simulink model "RM3_Hydraulic_PTO"  (R2019b)
settings: Solver=ode14x  StartTime=0  StopTime=100  FixedStep=0.0025  MaxStep=0.0025  RelTol=1e-3  EnableMultiTasking=on
undefined symbols (not defined in the file or in its folder): body, DiscIntNeverNeededParam, pto
libraries: fl_lib x208, sh_lib x67, nesl_utility x67, WECSim_Lib x5
(part 1 of 5)
settings Model: Creator=mlawson  LastModifiedBy=remil
settings SolverCC: ZeroCrossControl=DisableAll  AlgebraicLoopSolver=LineSearch  AutoInsertRateTranBlk=on
settings DataIOCC: SaveFormat=Array  SaveOutput=off  SaveTime=off  ReturnWorkspaceOutputs=off
settings OptimizationCC: LifeSpan=inf  SimCompilerOptimization=on
settings DebuggingCC: UnderspecifiedInitializationDetection=Classic  MergeDetectMultiDrivingBlocksExec=none  SolverPrmCheckMsg=warning  AllowSymbolicDim=off  StateNameClashWarn=warning  SFUnexpectedBacktrackingDiag=warning  SFNoUnconditionalDefaultTransitionDiag=warning  ArithmeticOperatorsInVariantConditions=warning
settings HardwareCC: ProdBitPerPointer=32  ProdBitPerSizeT=32  ProdBitPerPtrDiffT=32  ProdLargestAtomicFloat=None  ProdIntDivRoundTo=Undefined  ProdEndianess=Unspecified  ProdWordSize=32  ProdHWDeviceType=32-bit Generic
settings ModelReferenceCC: PropagateSignalLabelsOutOfModel=off
settings SFSimCC: SimUseLocalCustomCode=off  CustomCodeUndefinedFunction=UseInterfaceOnly
settings RTWCC: RTWUseLocalCustomCode=off
settings CodeAppCC: StateflowObjectComments=on
settings GRTTargetCC: TargetLangStandard=C89/C90 (ANSI)  GeneratePreprocessorConditionals=Disable all
settings ConfigComp: CovMetricSettings=dw  CovHtmlReporting=on  CovSaveCumulativeToWorkspaceVar=on  CovSaveSingleToWorkspaceVar=on  CovExternalEMLEnable=off  CovSFcnEnable=off
settings SimscapeCC: SimscapeNormalizeSystem=off  SimscapeLogType=all  SimscapeLogSimulationStatistics=on  SimscapeLogOpenViewer=on
settings SimMechanicsCC: VisDuringSimulation=on
settings ExplorerConfigSet: SimMechanicsOpenEditorOnUpdate=off

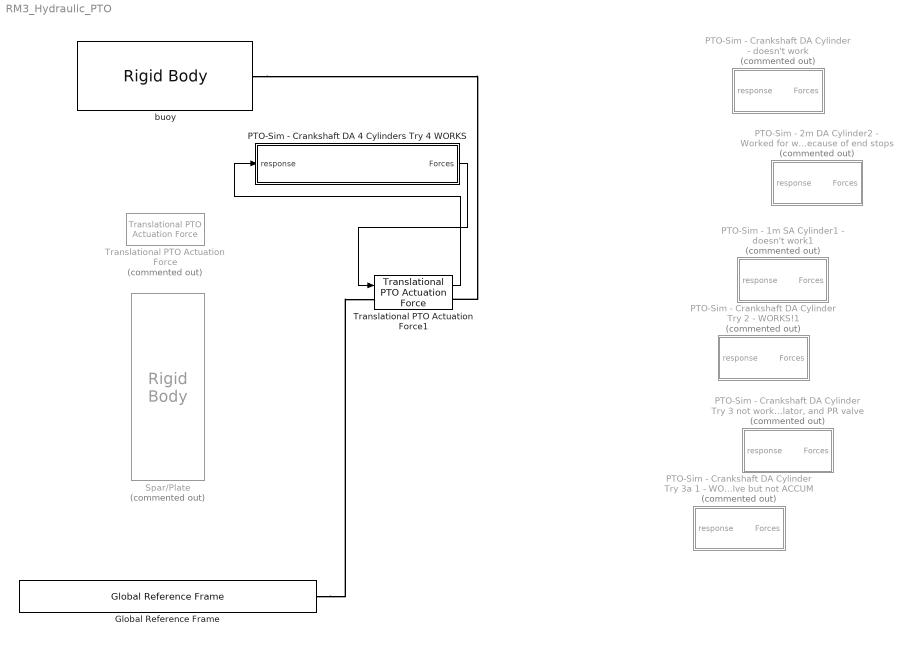
== system RM3_Hydraulic_PTO ==
  Global Reference Frame : WECSim_Lib/Frames/Global Reference Frame  waves=waves  simu=simu
      settings: SourceProductName=WEC-Sim
  PTO-Sim - 1m SA Cylinder1 - doesn't work1 : Subsystem  Commented=on
  "PTO-Sim - 2m DA Cylinder2 - Worked for waves up to 2m then forces go to infinity because of end stops   " : Subsystem  Commented=on
  "PTO-Sim - Crankshaft DA 4 Cylinders Try 4 WORKS " : Subsystem
  PTO-Sim - Crankshaft DA Cylinder - doesn't work : Subsystem  Commented=on
  PTO-Sim - Crankshaft DA Cylinder Try 2 - WORKS!1 : Subsystem  Commented=on
  "PTO-Sim - Crankshaft DA Cylinder Try 3 not working1 - added in correct PTO Force calculation, accumulator, and PR valve" : Subsystem  Commented=on
  PTO-Sim - Crankshaft DA Cylinder Try 3a 1 - WORKS - with PR valve but not ACCUM : Subsystem  Commented=on
  Spar/Plate : WECSim_Lib/Body Elements/Rigid Body  Commented=on  body=body(2)
      settings: AttributesFormatString=%<body>  SourceProductName=WEC-Sim
  Translational PTO Actuation Force : WECSim_Lib/PTOs/Translational PTO Actuation Force  Commented=on  pto=pto(1)
      settings: AttributesFormatString=%<pto>  SourceProductName=WEC-Sim
  Translational PTO Actuation Force1 : WECSim_Lib/PTOs/Translational PTO Actuation Force  pto=pto(1)
      settings: AttributesFormatString=%<pto>  SourceProductName=WEC-Sim
  buoy : WECSim_Lib/Body Elements/Rigid Body  body=body(1)
      settings: AttributesFormatString=%<body>  SourceProductName=WEC-Sim
  wires:
  "PTO-Sim - Crankshaft DA 4 Cylinders Try 4 WORKS "/1(Forces) -> Translational PTO Actuation Force1/1
  Translational PTO Actuation Force1/1 -> "PTO-Sim - Crankshaft DA 4 Cylinders Try 4 WORKS "/1(response)
  connections:
  buoy/RConn1 -- Translational PTO Actuation Force1/RConn1
  Global Reference Frame/RConn1 -- Translational PTO Actuation Force1/LConn1

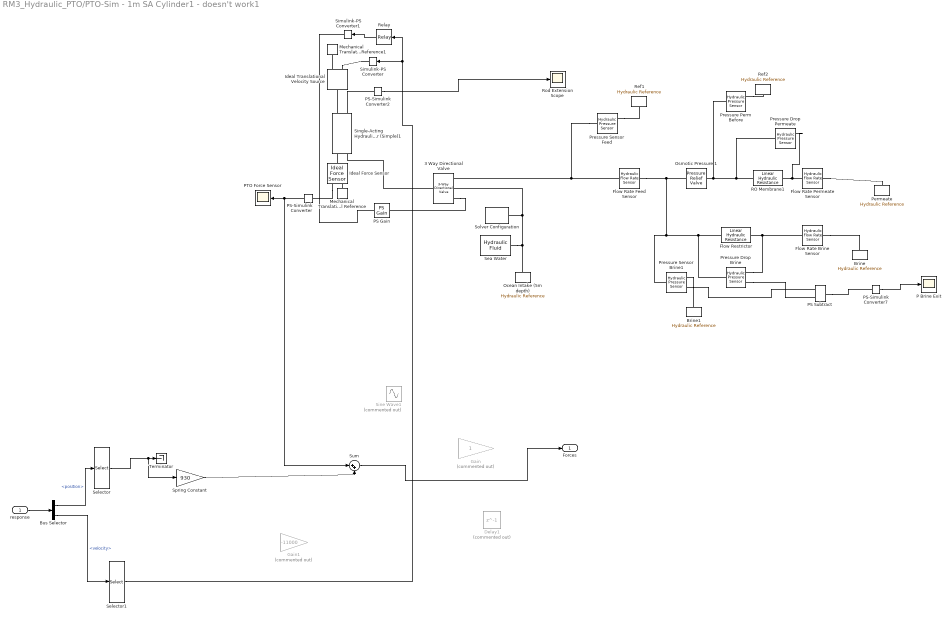
== system RM3_Hydraulic_PTO/PTO-Sim - 1m SA Cylinder1 - doesn't work1 ==
  response : Inport
  " Flow Rate Feed Sensor" : fl_lib/Hydraulic/Hydraulic Sensors/Hydraulic Flow Rate Sensor
      settings: SourceProductName=Simscape
  3 Way Directional Valve : sh_lib/Valves/Directional Valves/3-Way Directional Valve  area_spec=sh.valves.directional_valves.enum.area_spec.identical  x_0_P=0 m  x_0_T=0 m  mdl_type_identical=sh.valves.directional_valves.enum.mdl_type.linear  mdl_type_different=sh.valves.directional_valves.enum.mdl_type.linear  opening_max=0.75 in  area_max=pi*(0.75/2)^2 in^2  opening_max_P_A=0.005 m  area_max_P_A=0.5e-4 m^2  opening_max_A_T=0.005 m  area_max_A_T=0.5e-4 m^2  opening_area_tab=[-.002, 0, .002, .005, .015] m  area_tab=[1e-09, 2.0352e-07, 4.0736e-05, .00011438, .00034356] m^2  opening_flow_rate_tab=[-.002, 0, .002, .005, .015] m  pressure_tab=[-10000000, -5000000, -2000000, 2000000, 5000000, 10000000] Pa  flow_rate_tab=[-1e-07, -7.0711e-08, -4.4721e-08, 4.4721e-08, 7.0711e-08, 1e-07; -2.0352e-05, -1.4391e-05, -9.1017e-06, 9.1017e-06, 1.4391e-05, 2.0352e-05; -.0040736, -.0028805, -.0018218, .0018218, .0028805, .0040736; -.011438, -.0080879, -.0051152, .0051152, .0080879, .011438; -.034356, -.024293, -.015364, .015364, .024293, .034356] m^3/s  opening_area_tab_P_A=[-.002, 0, .002, .005, .015] m  area_tab_P_A=[1e-09, 2.0352e-07, 4.0736e-05, .00011438, .00034356] m^2  opening_flow_rate_tab_P_A=[-.002, 0, .002, .005, .015] m  pressure_tab_P_A=[-10000000, -5000000, -2000000, 2000000, 5000000, 10000000] Pa  flow_rate_tab_P_A=[-1e-07, -7.0711e-08, -4.4721e-08, 4.4721e-08, 7.0711e-08, 1e-07; -2.0352e-05, -1.4391e-05, -9.1017e-06, 9.1017e-06, 1.4391e-05, 2.0352e-05; -.0040736, -.0028805, -.0018218, .0018218, .0028805, .0040736; -.011438, -.0080879, -.0051152, .0051152, .0080879, .011438; -.034356, -.024293, -.015364, .015364, .024293, .034356] m^3/s  opening_area_tab_A_T=[-.002, 0, .002, .005, .015] m  area_tab_A_T=[1e-09, 2.0352e-07, 4.0736e-05, .00011438, .00034356] m^2  opening_flow_rate_tab_A_T=[-.002, 0, .002, .005, .015] m  pressure_tab_A_T=[-10000000, -5000000, -2000000, 2000000, 5000000, 10000000] Pa  flow_rate_tab_A_T=[-1e-07, -7.0711e-08, -4.4721e-08, 4.4721e-08, 7.0711e-08, 1e-07; -2.0352e-05, -1.4391e-05, -9.1017e-06, 9.1017e-06, 1.4391e-05, 2.0352e-05; -.0040736, -.0028805, -.0018218, .0018218, .0028805, .0040736; -.011438, -.0080879, -.0051152, .0051152, .0080879, .011438; -.034356, -.024293, -.015364, .015364, .024293, .034356] m^3/s  interp_method_identical=sh.valves.directional_valves.enum.interp_method.linear  interp_method_different=sh.valves.directional_valves.enum.interp_method.linear  extrap_method_identical=sh.valves.directional_valves.enum.extrap_method.linear  extrap_method_different=sh.valves.directional_valves.enum.extrap_method.linear  A_leak=1e-12 m^2  C_d=0.7  lam_spec=sh.valves.directional_valves.enum.lam_spec.pressure_ratio  B_lam=0.999  Re_cr=12
      settings: SourceProductName=Simscape Fluids  SourceProductBaseCode=SH  InternalSimscapePortConfiguration="{\"Bottom\":[],\"Left\":[{\"id\":\"A\",\"label\":\"A\",\"type\":\"foundation.hydraulic.hydraulic\"}],\"Right\":[{\"id\":\"S\",\"label\":\"S\",\"type\":\"input\"},{\"id\":\"P\",\"label\":\"P\",\"type\":\"foundation.hydraulic.hydraulic\"},{\"id\":\"T\",\"label\":\"T\",\"type\":\"foundation.hydraulic.hydraulic\"}],\"Top\":[]}"
  Brine : fl_lib/Hydraulic/Hydraulic Elements/Hydraulic Reference
      settings: SourceProductName=Simscape
  Brine1 : fl_lib/Hydraulic/Hydraulic Elements/Hydraulic Reference
      settings: SourceProductName=Simscape
  Bus Selector : BusSelector  OutputSignals=position,velocity
  Delay1 : Delay  Commented=on  DelayLength=1
  Flow Rate Brine Sensor : fl_lib/Hydraulic/Hydraulic Sensors/Hydraulic Flow Rate Sensor
      settings: SourceProductName=Simscape
  Flow Rate Permeate Sensor : fl_lib/Hydraulic/Hydraulic Sensors/Hydraulic Flow Rate Sensor
      settings: SourceProductName=Simscape
  Flow Restrictor : fl_lib/Hydraulic/Hydraulic Elements/Linear Hydraulic Resistance  resistance=(0.1) * ( 1/((3.812*10^-12)*(7.4 ) ) ) Pa/(m^3/s)  q_specify=off  q_priority=None  q=0.001 m^3/s  q_nominal_specify=off  q_nominal_unit=m^3/s  q_nominal_value=1  p_specify=off  p_priority=None  p=0 Pa  p_nominal_specify=off  p_nominal_unit=Pa  p_nominal_value=1
      settings: SourceProductName=Simscape  SourceProductBaseCode=SS  InternalSimscapePortConfiguration="{\"Bottom\":[],\"Left\":[{\"id\":\"A\",\"label\":\"A\",\"type\":\"foundation.hydraulic.hydraulic\"}],\"Right\":[{\"id\":\"B\",\"label\":\"B\",\"type\":\"foundation.hydraulic.hydraulic\"}],\"Top\":[]}"
  Gain : Gain  Commented=on
  Gain1 : Gain  Commented=on  Gain=-11000
  Ideal Force Sensor : fl_lib/Mechanical/Mechanical Sensors/Ideal Force Sensor
  Ideal Translational Velocity Source : fl_lib/Mechanical/Mechanical Sources/Ideal Translational Velocity Source
  Mechanical Translational Reference : fl_lib/Mechanical/Translational Elements/Mechanical Translational Reference
  Mechanical Translational Reference1 : fl_lib/Mechanical/Translational Elements/Mechanical Translational Reference
  Ocean Intake (5m depth) : fl_lib/Hydraulic/Hydraulic Elements/Hydraulic Reference
      settings: SourceProductName=Simscape
  Osmotic Pressure 1 : sh_lib/Valves/Pressure Control Valves/Pressure Relief Valve  valve_area_spec=1  p_diff_TLU=[30.15e5 : 15e3 : 31.35e5] Pa  area_TLU=[1 : 1 : 9] .* 1e-5 m^2  area_max=pi*(0.75/2)^2 in^2  pres_set=30 bar  reg_range=2 bar  C_d=0.7  A_leak=1e-12 m^2  lam_spec=1  B_lam=0.999  Re_cr=12  dynamic=0  tau=0.1 s  area_init=1e-12 m^2
      settings: SourceProductName=Simscape Fluids  SourceProductBaseCode=SH  InternalSimscapePortConfiguration="{\"Bottom\":[],\"Left\":[{\"id\":\"A\",\"label\":\"A\",\"type\":\"foundation.hydraulic.hydraulic\"}],\"Right\":[{\"id\":\"B\",\"label\":\"B\",\"type\":\"foundation.hydraulic.hydraulic\"}],\"Top\":[]}"
  P Brine Exit : Scope
  PS Gain : fl_lib/Physical Signals/Functions/PS Gain  gain=1
  PS Subtract : fl_lib/Physical Signals/Functions/PS Subtract
      settings: SourceProductName=Simscape
  PS-Simulink Converter : nesl_utility/PS-Simulink Converter  PhysicalDomain=network_engine_domain  SubClassName=ps_output  LeftPortType=input  RightPortType=output  PseudoPeriodic=off  Frequencies=[]  Unit=N  AffineConversion=off
  PS-Simulink Converter2 : nesl_utility/PS-Simulink Converter  PhysicalDomain=network_engine_domain  SubClassName=ps_output  LeftPortType=input  RightPortType=output  PseudoPeriodic=off  Frequencies=[]  Unit=m  AffineConversion=off
  PS-Simulink Converter7 : nesl_utility/PS-Simulink Converter  PhysicalDomain=network_engine_domain  SubClassName=ps_output  LeftPortType=input  RightPortType=output  PseudoPeriodic=off  Frequencies=[]  Unit=inherit  AffineConversion=off
  PTO Force Sensor : Scope
  Permeate : fl_lib/Hydraulic/Hydraulic Elements/Hydraulic Reference
      settings: SourceProductName=Simscape
  Pressure Drop Brine : fl_lib/Hydraulic/Hydraulic Sensors/Hydraulic Pressure Sensor
      settings: SourceProductName=Simscape
  Pressure Drop Permeate : fl_lib/Hydraulic/Hydraulic Sensors/Hydraulic Pressure Sensor
      settings: SourceProductName=Simscape
  Pressure Perm Before : fl_lib/Hydraulic/Hydraulic Sensors/Hydraulic Pressure Sensor
      settings: SourceProductName=Simscape
  Pressure Sensor Brine1 : fl_lib/Hydraulic/Hydraulic Sensors/Hydraulic Pressure Sensor
      settings: SourceProductName=Simscape
  Pressure Sensor Feed : fl_lib/Hydraulic/Hydraulic Sensors/Hydraulic Pressure Sensor
      settings: SourceProductName=Simscape
  RO Membrane1 : fl_lib/Hydraulic/Hydraulic Elements/Linear Hydraulic Resistance  resistance=1/((3.812*10^-12)*(7.4 ) ) Pa/(m^3/s)  q_specify=off  q_priority=None  q=0.001 m^3/s  q_nominal_specify=off  q_nominal_unit=m^3/s  q_nominal_value=1  p_specify=off  p_priority=None  p=0 Pa  p_nominal_specify=off  p_nominal_unit=Pa  p_nominal_value=1
      settings: SourceProductName=Simscape  SourceProductBaseCode=SS  InternalSimscapePortConfiguration="{\"Bottom\":[],\"Left\":[{\"id\":\"A\",\"label\":\"A\",\"type\":\"foundation.hydraulic.hydraulic\"}],\"Right\":[{\"id\":\"B\",\"label\":\"B\",\"type\":\"foundation.hydraulic.hydraulic\"}],\"Top\":[]}"
  Ref1 : fl_lib/Hydraulic/Hydraulic Elements/Hydraulic Reference
      settings: SourceProductName=Simscape
  Ref2 : fl_lib/Hydraulic/Hydraulic Elements/Hydraulic Reference
      settings: SourceProductName=Simscape
  Relay : Relay  OnSwitchValue=0  OffSwitchValue=0  OffOutputValue=-1
  Rod Extension Scope : Scope
  Sea Water : sh_lib/Hydraulic Utilities/Hydraulic Fluid  DataSource=1  SelFluid=24  SysTemp=30  TrapAir=0.005  ViscDerFactor=1  range_error=2
      settings: SourceProductName=Simscape Fluids
  Selector : Selector  InputPortWidth=6  IndexOptions=Index vector (dialog)  Indices=3  OutputSizes=1
  Selector1 : Selector  InputPortWidth=6  IndexOptions=Index vector (dialog)  Indices=3  OutputSizes=1
  Simulink-PS Converter : nesl_utility/Simulink-PS Converter  PhysicalDomain=network_engine_domain  SubClassName=ps_input  LeftPortType=input  RightPortType=output  PseudoPeriodic=off  Frequencies=[]  NoiseDistribution=none  NoiseParameters=[]  Unit=m/s  AffineConversion=off  FilteringAndDerivatives=filter  SimscapeFilterOrder=1  InputFilterTimeConstant=0.01  UdotUserProvided=0
  Simulink-PS Converter1 : nesl_utility/Simulink-PS Converter  PhysicalDomain=network_engine_domain  SubClassName=ps_input  LeftPortType=input  RightPortType=output  PseudoPeriodic=off  Frequencies=[]  NoiseDistribution=none  NoiseParameters=[]  Unit=1  AffineConversion=off  FilteringAndDerivatives=zero  SimscapeFilterOrder=1  InputFilterTimeConstant=0.001  UdotUserProvided=0
  Sine Wave1 : Sin  Commented=on  Amplitude=0.45/2  Frequency=0.9  SampleTime=0.01
  Single-Acting Hydraulic Cylinder (Simple)1 : sh_lib/Hydraulic Cylinders/Single-Acting Hydraulic Cylinder (Simple)  area=0.0025746658 m^2  stroke=1 m  init_pos=0.5 m  penetr_coeff=1e12 s*N/m^2  or=1
      settings: SourceProductName=Simscape Fluids  SourceProductBaseCode=SH  InternalSimscapePortConfiguration="{\"Bottom\":[],\"Left\":[{\"id\":\"C\",\"label\":\"C\",\"type\":\"foundation.mechanical.translational.translational\"},{\"id\":\"A\",\"label\":\"A\",\"type\":\"foundation.hydraulic.hydraulic\"}],\"Right\":[{\"id\":\"R\",\"label\":\"R\",\"type\":\"foundation.mechanical.translational.translational\"},{\"id\":\"P\",\"label\":\"P\",\"type\":\"output\"}],\"Top\":[]}"
  Solver Configuration : nesl_utility/Solver Configuration  PhysicalDomain=network_engine_domain  SubClassName=solver  LeftPortType=input  RightPortType=generic  Tones=[]  Harmonics=[]  SimulateNoise=off  Profile=off  UseLocalSampling=off  EnableSwitchedLinearOptims=on  FrequencyDomain=off  UseCCode=off  RelTol=0.001  AbsTol=1e-06  MinStep=1e-09  ToWorkspace=off  RevertToSquareIcSolve=off  NumHomotopyIterations=100  PhasorMode=off  PhasorModeNumHarmonics=1  DoDC=off  ResidualTolerance=1e-09  UseLocalSolver=off  LocalSolverChoice=NE_BACKWARD_EULER_ADVANCER  LocalSolverSampleTime=0.001  DoFixedCost=off  MaxNonlinIter=3  MaxModeIter=2  LinearAlgebra=auto  EquationFormulation=NE_TIME_EF  DelaysMemoryBudget=1024  AutomaticFiltering=on  FilteringTimeConstant=0.01  PartitionStorageMethod=AS_NEEDED  PartitionMemoryBudget=1024  PartitionMethod=ROBUST
  Spring Constant : Gain  Gain=930
  Sum : Sum  Inputs=|++
  Terminator : Terminator
  Forces : Outport  VectorParamsAs1DForOutWhenUnconnected=off
  wires:
  Bus Selector/1 -> Selector/1  "<position>"
  Bus Selector/2 -> Selector1/1  "<velocity>"
  response/1 -> Bus Selector/1
  Selector/1 -> Spring Constant/1, Terminator/1
  Sum/1 -> Forces/1
  PS-Simulink Converter2/1 -> Rod Extension Scope/1
  PS-Simulink Converter7/1 -> P Brine Exit/1
  Relay/1 -> Simulink-PS Converter1/1
  PS-Simulink Converter/1 -> Sum/1, PTO Force Sensor/1
  Spring Constant/1 -> Sum/2
  Selector1/1 -> Relay/1, Simulink-PS Converter/1
  connections:
  Pressure Drop Permeate/LConn1 -- RO Membrane1/LConn1 -- Osmotic Pressure 1/RConn1 -- Pressure Perm Before/LConn1
  Pressure Sensor Feed/LConn1 -- 3 Way Directional Valve/RConn3 -- " Flow Rate Feed Sensor"/LConn1
  Pressure Drop Permeate/RConn1 -- Flow Rate Permeate Sensor/LConn1 -- RO Membrane1/RConn1
  Pressure Sensor Brine1/LConn1 -- Flow Restrictor/LConn1 -- Pressure Drop Brine/LConn1 -- " Flow Rate Feed Sensor"/RConn2 -- Osmotic Pressure 1/LConn1
  Ocean Intake (5m depth)/LConn1 -- Solver Configuration/RConn1 -- 3 Way Directional Valve/RConn2 -- Sea Water/RConn1
  Pressure Drop Brine/RConn1 -- Flow Restrictor/RConn1 -- Flow Rate Brine Sensor/LConn1
  Simulink-PS Converter1/RConn1 -- PS Gain/LConn1
  Pressure Sensor Brine1/RConn1 -- Brine1/LConn1
  Single-Acting Hydraulic Cylinder (Simple)1/RConn1 -- Ideal Translational Velocity Source/LConn1
  Flow Rate Brine Sensor/RConn2 -- Brine/LConn1
  Pressure Perm Before/RConn1 -- Ref2/LConn1
  Pressure Drop Brine/RConn2 -- PS Subtract/LConn2
  Flow Rate Permeate Sensor/RConn2 -- Permeate/LConn1
  Ideal Force Sensor/LConn1 -- Single-Acting Hydraulic Cylinder (Simple)1/LConn1
  Single-Acting Hydraulic Cylinder (Simple)1/RConn2 -- PS-Simulink Converter2/LConn1
  PS Subtract/RConn1 -- PS-Simulink Converter7/LConn1
  Pressure Sensor Brine1/RConn2 -- PS Subtract/LConn1
  3 Way Directional Valve/LConn1 -- Single-Acting Hydraulic Cylinder (Simple)1/LConn2
  Ideal Force Sensor/RConn2 -- PS-Simulink Converter/LConn1
  Ideal Translational Velocity Source/RConn2 -- Mechanical Translational Reference1/LConn1
  Simulink-PS Converter/RConn1 -- Ideal Translational Velocity Source/RConn1
  Ideal Force Sensor/RConn1 -- Mechanical Translational Reference/LConn1
  3 Way Directional Valve/RConn1 -- PS Gain/RConn1
  Pressure Sensor Feed/RConn1 -- Ref1/LConn1

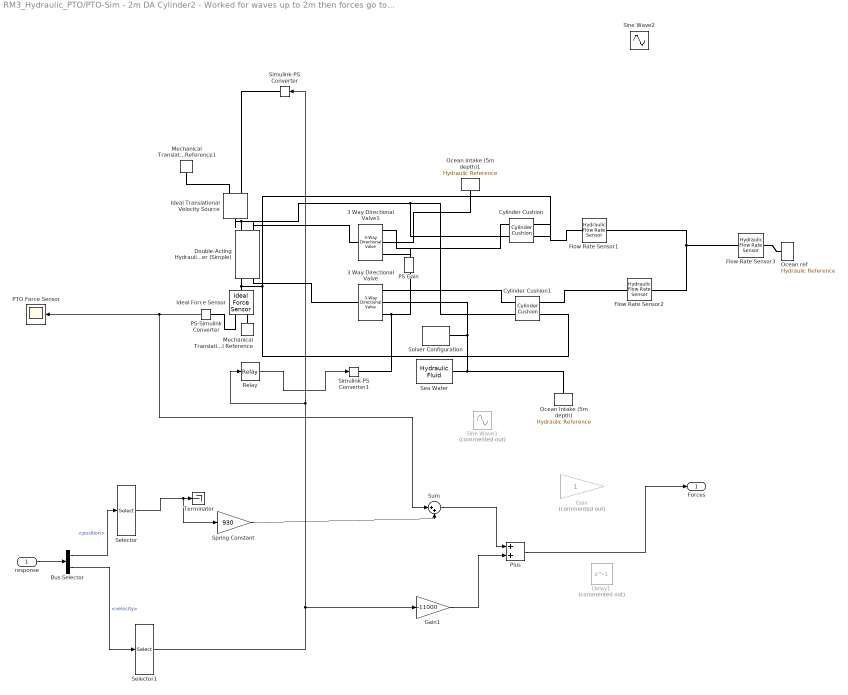
== system RM3_Hydraulic_PTO/PTO-Sim - 2m DA Cylinder2 - Worked for waves up to 2m then forces go to infinity because of end stops    ==
  response : Inport
  3 Way Directional Valve : sh_lib/Valves/Directional Valves/3-Way Directional Valve  area_spec=sh.valves.directional_valves.enum.area_spec.identical  x_0_P=0 m  x_0_T=0 m  mdl_type_identical=sh.valves.directional_valves.enum.mdl_type.linear  mdl_type_different=sh.valves.directional_valves.enum.mdl_type.linear  opening_max=0.75 in  area_max=pi*(0.75/2)^2 in^2  opening_max_P_A=0.005 m  area_max_P_A=0.5e-4 m^2  opening_max_A_T=0.005 m  area_max_A_T=0.5e-4 m^2  opening_area_tab=[-.002, 0, .002, .005, .015] m  area_tab=[1e-09, 2.0352e-07, 4.0736e-05, .00011438, .00034356] m^2  opening_flow_rate_tab=[-.002, 0, .002, .005, .015] m  pressure_tab=[-10000000, -5000000, -2000000, 2000000, 5000000, 10000000] Pa  flow_rate_tab=[-1e-07, -7.0711e-08, -4.4721e-08, 4.4721e-08, 7.0711e-08, 1e-07; -2.0352e-05, -1.4391e-05, -9.1017e-06, 9.1017e-06, 1.4391e-05, 2.0352e-05; -.0040736, -.0028805, -.0018218, .0018218, .0028805, .0040736; -.011438, -.0080879, -.0051152, .0051152, .0080879, .011438; -.034356, -.024293, -.015364, .015364, .024293, .034356] m^3/s  opening_area_tab_P_A=[-.002, 0, .002, .005, .015] m  area_tab_P_A=[1e-09, 2.0352e-07, 4.0736e-05, .00011438, .00034356] m^2  opening_flow_rate_tab_P_A=[-.002, 0, .002, .005, .015] m  pressure_tab_P_A=[-10000000, -5000000, -2000000, 2000000, 5000000, 10000000] Pa  flow_rate_tab_P_A=[-1e-07, -7.0711e-08, -4.4721e-08, 4.4721e-08, 7.0711e-08, 1e-07; -2.0352e-05, -1.4391e-05, -9.1017e-06, 9.1017e-06, 1.4391e-05, 2.0352e-05; -.0040736, -.0028805, -.0018218, .0018218, .0028805, .0040736; -.011438, -.0080879, -.0051152, .0051152, .0080879, .011438; -.034356, -.024293, -.015364, .015364, .024293, .034356] m^3/s  opening_area_tab_A_T=[-.002, 0, .002, .005, .015] m  area_tab_A_T=[1e-09, 2.0352e-07, 4.0736e-05, .00011438, .00034356] m^2  opening_flow_rate_tab_A_T=[-.002, 0, .002, .005, .015] m  pressure_tab_A_T=[-10000000, -5000000, -2000000, 2000000, 5000000, 10000000] Pa  flow_rate_tab_A_T=[-1e-07, -7.0711e-08, -4.4721e-08, 4.4721e-08, 7.0711e-08, 1e-07; -2.0352e-05, -1.4391e-05, -9.1017e-06, 9.1017e-06, 1.4391e-05, 2.0352e-05; -.0040736, -.0028805, -.0018218, .0018218, .0028805, .0040736; -.011438, -.0080879, -.0051152, .0051152, .0080879, .011438; -.034356, -.024293, -.015364, .015364, .024293, .034356] m^3/s  interp_method_identical=sh.valves.directional_valves.enum.interp_method.linear  interp_method_different=sh.valves.directional_valves.enum.interp_method.linear  extrap_method_identical=sh.valves.directional_valves.enum.extrap_method.linear  extrap_method_different=sh.valves.directional_valves.enum.extrap_method.linear  A_leak=1e-12 m^2  C_d=0.7  lam_spec=sh.valves.directional_valves.enum.lam_spec.pressure_ratio  B_lam=0.999  Re_cr=12
      settings: SourceProductName=Simscape Fluids  SourceProductBaseCode=SH  InternalSimscapePortConfiguration="{\"Bottom\":[],\"Left\":[{\"id\":\"A\",\"label\":\"A\",\"type\":\"foundation.hydraulic.hydraulic\"}],\"Right\":[{\"id\":\"S\",\"label\":\"S\",\"type\":\"input\"},{\"id\":\"P\",\"label\":\"P\",\"type\":\"foundation.hydraulic.hydraulic\"},{\"id\":\"T\",\"label\":\"T\",\"type\":\"foundation.hydraulic.hydraulic\"}],\"Top\":[]}"
  3 Way Directional Valve1 : sh_lib/Valves/Directional Valves/3-Way Directional Valve  area_spec=sh.valves.directional_valves.enum.area_spec.identical  x_0_P=0 m  x_0_T=0 m  mdl_type_identical=sh.valves.directional_valves.enum.mdl_type.linear  mdl_type_different=sh.valves.directional_valves.enum.mdl_type.linear  opening_max=0.75 in  area_max=pi*(0.75/2)^2 in^2  opening_max_P_A=0.005 m  area_max_P_A=0.5e-4 m^2  opening_max_A_T=0.005 m  area_max_A_T=0.5e-4 m^2  opening_area_tab=[-.002, 0, .002, .005, .015] m  area_tab=[1e-09, 2.0352e-07, 4.0736e-05, .00011438, .00034356] m^2  opening_flow_rate_tab=[-.002, 0, .002, .005, .015] m  pressure_tab=[-10000000, -5000000, -2000000, 2000000, 5000000, 10000000] Pa  flow_rate_tab=[-1e-07, -7.0711e-08, -4.4721e-08, 4.4721e-08, 7.0711e-08, 1e-07; -2.0352e-05, -1.4391e-05, -9.1017e-06, 9.1017e-06, 1.4391e-05, 2.0352e-05; -.0040736, -.0028805, -.0018218, .0018218, .0028805, .0040736; -.011438, -.0080879, -.0051152, .0051152, .0080879, .011438; -.034356, -.024293, -.015364, .015364, .024293, .034356] m^3/s  opening_area_tab_P_A=[-.002, 0, .002, .005, .015] m  area_tab_P_A=[1e-09, 2.0352e-07, 4.0736e-05, .00011438, .00034356] m^2  opening_flow_rate_tab_P_A=[-.002, 0, .002, .005, .015] m  pressure_tab_P_A=[-10000000, -5000000, -2000000, 2000000, 5000000, 10000000] Pa  flow_rate_tab_P_A=[-1e-07, -7.0711e-08, -4.4721e-08, 4.4721e-08, 7.0711e-08, 1e-07; -2.0352e-05, -1.4391e-05, -9.1017e-06, 9.1017e-06, 1.4391e-05, 2.0352e-05; -.0040736, -.0028805, -.0018218, .0018218, .0028805, .0040736; -.011438, -.0080879, -.0051152, .0051152, .0080879, .011438; -.034356, -.024293, -.015364, .015364, .024293, .034356] m^3/s  opening_area_tab_A_T=[-.002, 0, .002, .005, .015] m  area_tab_A_T=[1e-09, 2.0352e-07, 4.0736e-05, .00011438, .00034356] m^2  opening_flow_rate_tab_A_T=[-.002, 0, .002, .005, .015] m  pressure_tab_A_T=[-10000000, -5000000, -2000000, 2000000, 5000000, 10000000] Pa  flow_rate_tab_A_T=[-1e-07, -7.0711e-08, -4.4721e-08, 4.4721e-08, 7.0711e-08, 1e-07; -2.0352e-05, -1.4391e-05, -9.1017e-06, 9.1017e-06, 1.4391e-05, 2.0352e-05; -.0040736, -.0028805, -.0018218, .0018218, .0028805, .0040736; -.011438, -.0080879, -.0051152, .0051152, .0080879, .011438; -.034356, -.024293, -.015364, .015364, .024293, .034356] m^3/s  interp_method_identical=sh.valves.directional_valves.enum.interp_method.linear  interp_method_different=sh.valves.directional_valves.enum.interp_method.linear  extrap_method_identical=sh.valves.directional_valves.enum.extrap_method.linear  extrap_method_different=sh.valves.directional_valves.enum.extrap_method.linear  A_leak=1e-12 m^2  C_d=0.7  lam_spec=sh.valves.directional_valves.enum.lam_spec.pressure_ratio  B_lam=0.999  Re_cr=12
      settings: SourceProductName=Simscape Fluids  SourceProductBaseCode=SH  InternalSimscapePortConfiguration="{\"Bottom\":[],\"Left\":[{\"id\":\"A\",\"label\":\"A\",\"type\":\"foundation.hydraulic.hydraulic\"}],\"Right\":[{\"id\":\"S\",\"label\":\"S\",\"type\":\"input\"},{\"id\":\"P\",\"label\":\"P\",\"type\":\"foundation.hydraulic.hydraulic\"},{\"id\":\"T\",\"label\":\"T\",\"type\":\"foundation.hydraulic.hydraulic\"}],\"Top\":[]}"
  Bus Selector : BusSelector  OutputSignals=position,velocity
  Cylinder Cushion : sh_lib/Hydraulic Cylinders/Cylinder Cushion  piston_area=0.0025746658 m^2  piston_init_pos=1 m  orient=1  orifice_area=1e-6 m^2  orifice_C_d=0.7  orifice_Re=10  check_area=1e-4 m^2  check_cr_pr=0.5e5 Pa  check_op_pr=1.5e5 Pa  check_C_d=0.7  check_Re=10  check_leak_area=1e-12 m^2  opening="[-2,       10,    11,   20,    89,      90,    102] mm"  area=[.002, .006, .020, 9*10, 9*10, 9*10, 9*10] cm^2  var_orif_interp=1  var_orif_extrap=1  var_orif_C_d=0.7  var_orif_Re=10  var_orif_leak=1e-12 m^2
      settings: SourceProductName=Simscape Fluids  SourceProductBaseCode=SH  InternalSimscapePortConfiguration="{\"Bottom\":[],\"Left\":[{\"id\":\"C\",\"label\":\"C\",\"type\":\"foundation.mechanical.translational.translational\"},{\"id\":\"A\",\"label\":\"A\",\"type\":\"foundation.hydraulic.hydraulic\"}],\"Right\":[{\"id\":\"R\",\"label\":\"R\",\"type\":\"foundation.mechanical.translational.translational\"},{\"id\":\"B\",\"label\":\"B\",\"type\":\"foundation.hydraulic.hydraulic\"}],\"Top\":[]}"
  Cylinder Cushion1 : sh_lib/Hydraulic Cylinders/Cylinder Cushion  piston_area=0.0025746658 m^2  piston_init_pos=1 m  orient=1  orifice_area=1e-6 m^2  orifice_C_d=0.7  orifice_Re=10  check_area=1e-4 m^2  check_cr_pr=0.5e5 Pa  check_op_pr=1.5e5 Pa  check_C_d=0.7  check_Re=10  check_leak_area=1e-12 m^2  opening="[-2,       10,    11,   20,    89,      90,    102] mm"  area=[.002, .006, .020, 9*10, 9*10, 9*10, 9*10] cm^2  var_orif_interp=1  var_orif_extrap=1  var_orif_C_d=0.7  var_orif_Re=10  var_orif_leak=1e-12 m^2
      settings: SourceProductName=Simscape Fluids  SourceProductBaseCode=SH  InternalSimscapePortConfiguration="{\"Bottom\":[],\"Left\":[{\"id\":\"C\",\"label\":\"C\",\"type\":\"foundation.mechanical.translational.translational\"},{\"id\":\"A\",\"label\":\"A\",\"type\":\"foundation.hydraulic.hydraulic\"}],\"Right\":[{\"id\":\"R\",\"label\":\"R\",\"type\":\"foundation.mechanical.translational.translational\"},{\"id\":\"B\",\"label\":\"B\",\"type\":\"foundation.hydraulic.hydraulic\"}],\"Top\":[]}"
  Delay1 : Delay  Commented=on  DelayLength=1
  Double-Acting Hydraulic Cylinder (Simple) : sh_lib/Hydraulic Cylinders/Double-Acting Hydraulic Cylinder (Simple)  area_A=0.0025746658 m^2  area_B=0.0025746658 m^2  stroke=2 m  init_pos=1 m  penetr_coeff=1e12 s*N/m^2  or=1
      settings: SourceProductName=Simscape Fluids  SourceProductBaseCode=SH  InternalSimscapePortConfiguration="{\"Bottom\":[],\"Left\":[{\"id\":\"C\",\"label\":\"C\",\"type\":\"foundation.mechanical.translational.translational\"},{\"id\":\"A\",\"label\":\"A\",\"type\":\"foundation.hydraulic.hydraulic\"}],\"Right\":[{\"id\":\"R\",\"label\":\"R\",\"type\":\"foundation.mechanical.translational.translational\"},{\"id\":\"B\",\"label\":\"B\",\"type\":\"foundation.hydraulic.hydraulic\"}],\"Top\":[]}"
  Flow Rate Sensor1 : fl_lib/Hydraulic/Hydraulic Sensors/Hydraulic Flow Rate Sensor
      settings: SourceProductName=Simscape
  Flow Rate Sensor2 : fl_lib/Hydraulic/Hydraulic Sensors/Hydraulic Flow Rate Sensor
      settings: SourceProductName=Simscape
  Flow Rate Sensor3 : fl_lib/Hydraulic/Hydraulic Sensors/Hydraulic Flow Rate Sensor
      settings: SourceProductName=Simscape
  Gain : Gain  Commented=on
  Gain1 : Gain  Gain=-11000
  Ideal Force Sensor : fl_lib/Mechanical/Mechanical Sensors/Ideal Force Sensor
  Ideal Translational Velocity Source : fl_lib/Mechanical/Mechanical Sources/Ideal Translational Velocity Source
  Mechanical Translational Reference : fl_lib/Mechanical/Translational Elements/Mechanical Translational Reference
  Mechanical Translational Reference1 : fl_lib/Mechanical/Translational Elements/Mechanical Translational Reference
  Ocean Intake (5m depth) : fl_lib/Hydraulic/Hydraulic Elements/Hydraulic Reference
      settings: SourceProductName=Simscape
  Ocean Intake (5m depth)1 : fl_lib/Hydraulic/Hydraulic Elements/Hydraulic Reference
      settings: SourceProductName=Simscape
  "Ocean ref " : fl_lib/Hydraulic/Hydraulic Elements/Hydraulic Reference
      settings: SourceProductName=Simscape
  PS Gain : fl_lib/Physical Signals/Functions/PS Gain  gain=-1
  PS-Simulink Converter : nesl_utility/PS-Simulink Converter  PhysicalDomain=network_engine_domain  SubClassName=ps_output  LeftPortType=input  RightPortType=output  PseudoPeriodic=off  Frequencies=[]  Unit=N  AffineConversion=off
  PTO Force Sensor : Scope
  Plus : Sum
  Relay : Relay  OnSwitchValue=0  OffSwitchValue=0  OffOutputValue=-1
  Sea Water : sh_lib/Hydraulic Utilities/Hydraulic Fluid  DataSource=1  SelFluid=24  SysTemp=30  TrapAir=0.005  ViscDerFactor=1  range_error=2
      settings: SourceProductName=Simscape Fluids
  Selector : Selector  InputPortWidth=6  IndexOptions=Index vector (dialog)  Indices=3  OutputSizes=1
  Selector1 : Selector  InputPortWidth=6  IndexOptions=Index vector (dialog)  Indices=3  OutputSizes=1
  Simulink-PS Converter : nesl_utility/Simulink-PS Converter  PhysicalDomain=network_engine_domain  SubClassName=ps_input  LeftPortType=input  RightPortType=output  PseudoPeriodic=off  Frequencies=[]  NoiseDistribution=none  NoiseParameters=[]  Unit=m/s  AffineConversion=off  FilteringAndDerivatives=filter  SimscapeFilterOrder=2  InputFilterTimeConstant=0.01  UdotUserProvided=0
  Simulink-PS Converter1 : nesl_utility/Simulink-PS Converter  PhysicalDomain=network_engine_domain  SubClassName=ps_input  LeftPortType=input  RightPortType=output  PseudoPeriodic=off  Frequencies=[]  NoiseDistribution=none  NoiseParameters=[]  Unit=1  AffineConversion=off  FilteringAndDerivatives=filter  SimscapeFilterOrder=1  InputFilterTimeConstant=0.01  UdotUserProvided=0
  Sine Wave1 : Sin  Commented=on  Amplitude=0.45/2  Frequency=0.9  SampleTime=0.01
  Sine Wave2 : Sin  Amplitude=0.45  Frequency=0.9  Phase=pi/2  SampleTime=0.01
  Solver Configuration : nesl_utility/Solver Configuration  PhysicalDomain=network_engine_domain  SubClassName=solver  LeftPortType=input  RightPortType=generic  Tones=[]  Harmonics=[]  SimulateNoise=off  Profile=off  UseLocalSampling=off  EnableSwitchedLinearOptims=on  FrequencyDomain=off  UseCCode=off  RelTol=0.001  AbsTol=1e-06  MinStep=1e-09  ToWorkspace=off  RevertToSquareIcSolve=off  NumHomotopyIterations=100  PhasorMode=off  PhasorModeNumHarmonics=1  DoDC=off  ResidualTolerance=1e-09  UseLocalSolver=off  LocalSolverChoice=NE_BACKWARD_EULER_ADVANCER  LocalSolverSampleTime=0.001  DoFixedCost=off  MaxNonlinIter=3  MaxModeIter=2  LinearAlgebra=auto  EquationFormulation=NE_TIME_EF  DelaysMemoryBudget=1024  AutomaticFiltering=on  FilteringTimeConstant=0.01  PartitionStorageMethod=AS_NEEDED  PartitionMemoryBudget=1024  PartitionMethod=ROBUST
  Spring Constant : Gain  Gain=930
  Sum : Sum  Inputs=|++
  Terminator : Terminator
  Forces : Outport  VectorParamsAs1DForOutWhenUnconnected=off
  wires:
  Bus Selector/1 -> Selector/1  "<position>"
  Bus Selector/2 -> Selector1/1  "<velocity>"
  response/1 -> Bus Selector/1
  Selector/1 -> Spring Constant/1, Terminator/1
  Sum/1 -> Plus/1
  Spring Constant/1 -> Sum/2
  Relay/1 -> Simulink-PS Converter1/1
  PS-Simulink Converter/1 -> Sum/1, PTO Force Sensor/1
  Selector1/1 -> Gain1/1, Relay/1, Simulink-PS Converter/1
  Gain1/1 -> Plus/2
  Plus/1 -> Forces/1
  connections:
  3 Way Directional Valve/RConn1 -- Simulink-PS Converter1/RConn1 -- PS Gain/LConn1
  Cylinder Cushion1/RConn1 -- Double-Acting Hydraulic Cylinder (Simple)/RConn1 -- Ideal Translational Velocity Source/LConn1 -- Cylinder Cushion/RConn1
  Double-Acting Hydraulic Cylinder (Simple)/LConn1 -- Ideal Force Sensor/LConn1 -- Cylinder Cushion/LConn1 -- Cylinder Cushion1/LConn1
  Flow Rate Sensor3/LConn1 -- Flow Rate Sensor1/RConn2 -- Flow Rate Sensor2/RConn2
  Solver Configuration/RConn1 -- Ocean Intake (5m depth)/LConn1 -- Sea Water/RConn1 -- 3 Way Directional Valve/RConn2
  3 Way Directional Valve/LConn1 -- Double-Acting Hydraulic Cylinder (Simple)/LConn2
  Flow Rate Sensor1/LConn1 -- Cylinder Cushion/LConn2
  Ideal Translational Velocity Source/RConn2 -- Mechanical Translational Reference1/LConn1
  Double-Acting Hydraulic Cylinder (Simple)/RConn2 -- 3 Way Directional Valve1/LConn1
  Ideal Force Sensor/RConn1 -- Mechanical Translational Reference/LConn1
  Flow Rate Sensor3/RConn2 -- "Ocean ref "/LConn1
  Ideal Force Sensor/RConn2 -- PS-Simulink Converter/LConn1
  Ideal Translational Velocity Source/RConn1 -- Simulink-PS Converter/RConn1
  PS Gain/RConn1 -- 3 Way Directional Valve1/RConn1
  Cylinder Cushion1/LConn2 -- Flow Rate Sensor2/LConn1
  Cylinder Cushion/RConn2 -- 3 Way Directional Valve1/RConn3
  3 Way Directional Valve/RConn3 -- Cylinder Cushion1/RConn2
  Ocean Intake (5m depth)1/LConn1 -- 3 Way Directional Valve1/RConn2

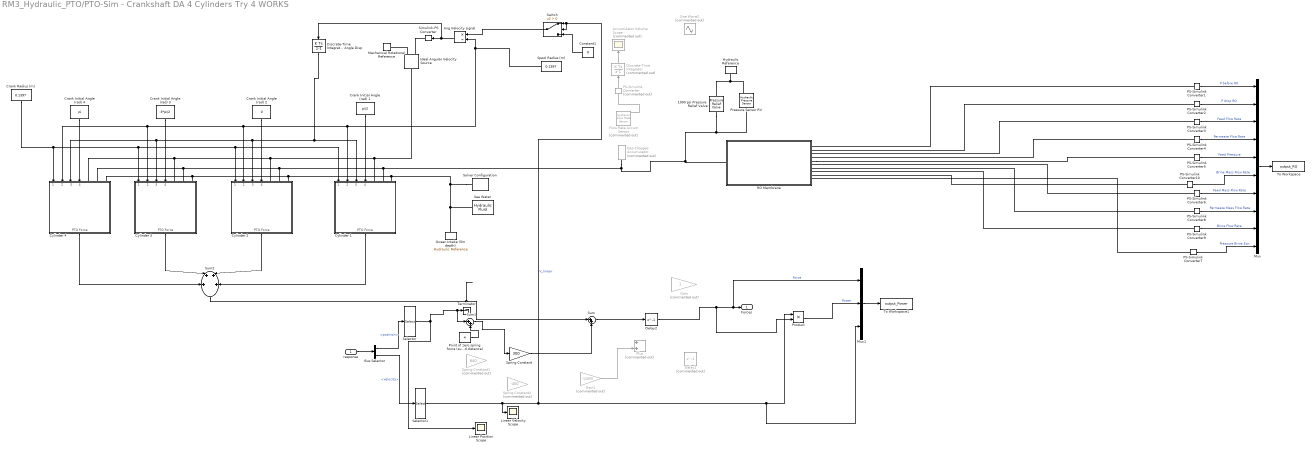
== system RM3_Hydraulic_PTO/PTO-Sim - Crankshaft DA 4 Cylinders Try 4 WORKS  ==
  response : Inport
  " Flow Rate Accum Sensor" : fl_lib/Hydraulic/Hydraulic Sensors/Hydraulic Flow Rate Sensor  Commented=on
      settings: SourceProductName=Simscape
  1000 psi Pressure Relief Valve : sh_lib/Valves/Pressure Control Valves/Pressure Relief Valve  valve_area_spec=1  p_diff_TLU=[30.15e5 : 15e3 : 31.35e5] Pa  area_TLU=[1 : 1 : 9] .* 1e-5 m^2  area_max=pi*(0.75/2)^2 in^2  pres_set=1000 psi  reg_range=50 psi  C_d=0.7  A_leak=1e-12 m^2  lam_spec=1  B_lam=0.999  Re_cr=12  dynamic=0  tau=0.1 s  area_init=1e-12 m^2
      settings: SourceProductName=Simscape Fluids  SourceProductBaseCode=SH  InternalSimscapePortConfiguration="{\"Bottom\":[],\"Left\":[{\"id\":\"A\",\"label\":\"A\",\"type\":\"foundation.hydraulic.hydraulic\"}],\"Right\":[{\"id\":\"B\",\"label\":\"B\",\"type\":\"foundation.hydraulic.hydraulic\"}],\"Top\":[]}"
  Accumulator Volume Scope : Scope  Commented=on
  Ang Velocity signal : Product  Inputs=*/
  Bus Selector : BusSelector  OutputSignals=position,velocity
  Constant1 : Constant  Value=0
  Crank Initial Angle (rad) 1 : Constant  Value=pi/2
  Crank Initial Angle (rad) 2 : Constant  Value=0
  Crank Initial Angle (rad) 3 : Constant  Value=3*pi/2
  Crank Initial Angle (rad) 4 : Constant  Value=pi
  Crank Radius (m) : Constant  Value=0.1397
  Cylinder 1 : Subsystem
  Cylinder 2 : Subsystem
  Cylinder 3 : Subsystem
  Cylinder 4 : Subsystem
  Delay1 : Delay  Commented=on  DelayLength=1
  Delay2 : Delay  DelayLength=1
  Discrete-Time Integrator : DiscreteIntegrator  Commented=on  SampleTime=-1  ICPrevOutput=DiscIntNeverNeededParam  ICPrevScaledInput=DiscIntNeverNeededParam
  Discrete-Time Integrator - Angle Disp : DiscreteIntegrator  SampleTime=-1  ICPrevOutput=DiscIntNeverNeededParam  ICPrevScaledInput=DiscIntNeverNeededParam
  Gain : Gain  Commented=on
  Gain1 : Gain  Commented=on  Gain=-11000
  Gas-Charged Accumulator : sh_lib/Accumulators/Gas-Charged Accumulator  Commented=on  capacity=2.5 gal  dead_volume=4e-5 m^3  pr_preload=800 psi  k_sh=1.4  stiff_coeff=1e10 Pa/m^3  penetr_coeff=1e10 s*Pa/m^6  flow_rate_specify=off  flow_rate_priority=None  flow_rate=0.005 m^3/s  flow_rate_nominal_specify=off  flow_rate_nominal_unit=m^3/s  flow_rate_nominal_value=1  liquid_volume_specify=on  liquid_volume_priority=High  liquid_volume=0.005 m^3  liquid_volume_nominal_specify=off  liquid_volume_nominal_unit=m^3  liquid_volume_nominal_value=1  liquid_pressure_specify=off  liquid_pressure_priority=None  liquid_pressure=1.01325e+5 Pa  liquid_pressure_nominal_specify=off  liquid_pressure_nominal_unit=Pa  liquid_pressure_nominal_value=1
      settings: SourceProductName=Simscape Fluids  SourceProductBaseCode=SH  InternalSimscapePortConfiguration="{\"Bottom\":[],\"Left\":[],\"Right\":[{\"id\":\"A\",\"label\":\"A\",\"type\":\"foundation.hydraulic.hydraulic\"}],\"Top\":[]}"
  Hydraulic Reference : fl_lib/Hydraulic/Hydraulic Elements/Hydraulic Reference
      settings: SourceProductName=Simscape
  Ideal Angular Velocity Source : fl_lib/Mechanical/Mechanical Sources/Ideal Angular Velocity Source
  Linear Position Scope : Scope
  Linear Velocity Scope : Scope
  Mechanical Rotational Reference : fl_lib/Mechanical/Rotational Elements/Mechanical Rotational Reference
  Mux : Mux  Inputs=10
  Mux1 : Mux  Inputs=3
  Ocean Intake (5m depth) : fl_lib/Hydraulic/Hydraulic Elements/Hydraulic Reference
      settings: SourceProductName=Simscape
  PS-Simulink Converter : nesl_utility/PS-Simulink Converter  Commented=on  PhysicalDomain=network_engine_domain  SubClassName=ps_output  LeftPortType=input  RightPortType=output  PseudoPeriodic=off  Frequencies=[]  Unit=inherit  AffineConversion=off
  PS-Simulink Converter{1..10} (10 alike) : nesl_utility/PS-Simulink Converter  PhysicalDomain=network_engine_domain  SubClassName=ps_output  LeftPortType=input  RightPortType=output  PseudoPeriodic=off  Frequencies=[]  Unit=inherit  AffineConversion=off
  Plus : Sum  Commented=on
  "Point of zero spring force (submerged distance) " : Constant  Value=4
  Pressure Sensor RV : fl_lib/Hydraulic/Hydraulic Sensors/Hydraulic Pressure Sensor
      settings: SourceProductName=Simscape
  Product : Product
  RO Membrane : Subsystem
  Sea Water : sh_lib/Hydraulic Utilities/Hydraulic Fluid  DataSource=1  SelFluid=24  SysTemp=30  TrapAir=0.005  ViscDerFactor=1  range_error=2
      settings: SourceProductName=Simscape Fluids
  Selector : Selector  InputPortWidth=6  IndexOptions=Index vector (dialog)  Indices=3  OutputSizes=1
  Selector1 : Selector  InputPortWidth=6  IndexOptions=Index vector (dialog)  Indices=3  OutputSizes=1
  Simulink-PS Converter : nesl_utility/Simulink-PS Converter  PhysicalDomain=network_engine_domain  SubClassName=ps_input  LeftPortType=input  RightPortType=output  PseudoPeriodic=off  Frequencies=[]  NoiseDistribution=none  NoiseParameters=[]  Unit=rad/s  AffineConversion=off  FilteringAndDerivatives=filter  SimscapeFilterOrder=2  InputFilterTimeConstant=0.001  UdotUserProvided=0
  Sine Wave2 : Sin  Commented=on  Amplitude=0.45  Frequency=0.9  SampleTime=0.01
  Solver Configuration : nesl_utility/Solver Configuration  PhysicalDomain=network_engine_domain  SubClassName=solver  LeftPortType=input  RightPortType=generic  Tones=[]  Harmonics=[]  SimulateNoise=off  Profile=off  UseLocalSampling=off  EnableSwitchedLinearOptims=on  FrequencyDomain=off  UseCCode=off  RelTol=0.001  AbsTol=1e-06  MinStep=1e-09  ToWorkspace=off  RevertToSquareIcSolve=off  NumHomotopyIterations=100  PhasorMode=off  PhasorModeNumHarmonics=1  DoDC=off  ResidualTolerance=1e-09  UseLocalSolver=off  LocalSolverChoice=NE_BACKWARD_EULER_ADVANCER  LocalSolverSampleTime=0.001  DoFixedCost=off  MaxNonlinIter=3  MaxModeIter=2  LinearAlgebra=auto  EquationFormulation=NE_TIME_EF  DelaysMemoryBudget=1024  AutomaticFiltering=on  FilteringTimeConstant=0.01  PartitionStorageMethod=AS_NEEDED  PartitionMemoryBudget=1024  PartitionMethod=ROBUST
  Spool Radius (m) : Constant  Value=0.1397
  Spring Constant : Gain  Gain=300
  Spring Constant1 : Gain  Commented=on  Gain=840
  Spring Constant2 : Gain  Commented=on  Gain=-400
  Sum : Sum  Inputs=|++
  Sum1 : Sum  Inputs=|++
  Sum2 : Sum  Inputs=4
  Switch : Switch  Criteria=u2 > Threshold
  Terminator : Terminator
  To Workspace : ToWorkspace  VariableName=output_RO  SaveFormat=Structure With Time  SampleTime=-1
  To Workspace1 : ToWorkspace  VariableName=output_Power  SaveFormat=Structure With Time  SampleTime=-1
  Forces : Outport  VectorParamsAs1DForOutWhenUnconnected=off
  wires:
  Bus Selector/1 -> Selector/1  "<position>"
  Bus Selector/2 -> Selector1/1  "<velocity>"
  response/1 -> Bus Selector/1
  Selector/1 -> Linear Position Scope/1, Sum1/1, Terminator/1
  Spring Constant/1 -> Sum/2
  Gain1/1 -> Plus/2
  Sum/1 -> Delay2/1
  Constant1/1 -> Switch/3
  Switch/1 -> Ang Velocity signal/1
  Selector1/1 -> Linear Velocity Scope/1, Mux1/3, Product/1, Switch/2, Switch/1  "V_linear"
  Ang Velocity signal/1 -> Discrete-Time Integrator - Angle Disp/1, Simulink-PS Converter/1
  "Point of zero spring force (submerged distance) "/1 -> Sum1/2
  Sum1/1 -> Spring Constant/1
  Delay2/1 -> Product/2, Mux1/1, Forces/1  "Force"
  PS-Simulink Converter/1 -> Discrete-Time Integrator/1
  Discrete-Time Integrator/1 -> Accumulator Volume Scope/1
  Crank Radius (m)/1 -> Cylinder 4/1(Crank Radius), Cylinder 3/1(Crank Radius), Cylinder 2/1(Crank Radius), Cylinder 1/1(Crank Radius)
  Discrete-Time Integrator - Angle Disp/1 -> Cylinder 4/3(Angle Displacement), Cylinder 3/3(Angle Displacement), Cylinder 2/3(Angle Displacement), Cylinder 1/3(Angle Displacement)
  Crank Initial Angle (rad) 1/1 -> Cylinder 1/4(Crank Init Angle)
  Sum2/1 -> Sum/1
  Cylinder 1/1(PTO Force) -> Sum2/4
  Cylinder 2/1(PTO Force) -> Sum2/3
  Cylinder 3/1(PTO Force) -> Sum2/2
  Cylinder 4/1(PTO Force) -> Sum2/1
  Spool Radius (m)/1 -> Cylinder 1/2(Spool Radius), Cylinder 4/2(Spool Radius), Cylinder 3/2(Spool Radius), Cylinder 2/2(Spool Radius), Ang Velocity signal/2
  Crank Initial Angle (rad) 4/1 -> Cylinder 4/4(Crank Init Angle)
  Crank Initial Angle (rad) 3/1 -> Cylinder 3/4(Crank Init Angle)
  Crank Initial Angle (rad) 2/1 -> Cylinder 2/4(Crank Init Angle)
  PS-Simulink Converter6/1 -> Mux/7  "Feed Mass Flow Rate"
  PS-Simulink Converter10/1 -> Mux/6  "Brine Mass Flow Rate"
  PS-Simulink Converter9/1 -> Mux/9  "Brine Flow Rate"
  PS-Simulink Converter8/1 -> Mux/8  "Permeate Mass Flow Rate"
  Mux/1 -> To Workspace/1
  PS-Simulink Converter4/1 -> Mux/4  "Permeate Flow Rate"
  PS-Simulink Converter1/1 -> Mux/1  "P before RO"
  PS-Simulink Converter2/1 -> Mux/2  "P drop RO"
  PS-Simulink Converter3/1 -> Mux/3  "Feed Flow Rate"
  PS-Simulink Converter5/1 -> Mux/5  "Feed Pressure"
  PS-Simulink Converter7/1 -> Mux/10  "Pressure Brine Exit"
  Mux1/1 -> To Workspace1/1
  Product/1 -> Mux1/2  "Power"
  connections:
  Solver Configuration/RConn1 -- Ocean Intake (5m depth)/LConn1 -- Sea Water/RConn1 -- Cylinder 4/LConn3 -- Cylinder 3/LConn3 -- Cylinder 2/LConn3 -- Cylinder 1/LConn3
  Ideal Angular Velocity Source/RConn2 -- Mechanical Rotational Reference/LConn1
  Ideal Angular Velocity Source/RConn1 -- Simulink-PS Converter/RConn1
  1000 psi Pressure Relief Valve/RConn1 -- Pressure Sensor RV/RConn1 -- Hydraulic Reference/LConn1
  Gas-Charged Accumulator/RConn1 -- Cylinder 1/LConn2 -- Cylinder 3/LConn2 -- Cylinder 4/LConn2 -- Cylinder 2/LConn2 -- RO Membrane/LConn1 -- 1000 psi Pressure Relief Valve/LConn1 -- Pressure Sensor RV/LConn1
  " Flow Rate Accum Sensor"/RConn1 -- PS-Simulink Converter/LConn1
  Cylinder 1/LConn1 -- Cylinder 2/LConn1 -- Cylinder 3/LConn1 -- Cylinder 4/LConn1 -- Ideal Angular Velocity Source/LConn1
  PS-Simulink Converter10/LConn1 -- RO Membrane/RConn9
  PS-Simulink Converter3/LConn1 -- RO Membrane/RConn3
  PS-Simulink Converter9/LConn1 -- RO Membrane/RConn8
  PS-Simulink Converter1/LConn1 -- RO Membrane/RConn1
  PS-Simulink Converter8/LConn1 -- RO Membrane/RConn7
  PS-Simulink Converter6/LConn1 -- RO Membrane/RConn6
  PS-Simulink Converter4/LConn1 -- RO Membrane/RConn4
  PS-Simulink Converter2/LConn1 -- RO Membrane/RConn2
  RO Membrane/RConn5 -- PS-Simulink Converter5/LConn1
  PS-Simulink Converter7/LConn1 -- RO Membrane/RConn10
